simulink model "PlantModel"  (R2021b)
settings: configuration reference "MIL_Simulation_ConfigSet" (kept outside this file)
PreLoadFcn:
  | run_start;
undefined symbols (not defined in the file or in its folder): DiscIntNeverNeededParam, F, inverter_ena, J, L_d, L_q, p, Psi_p, R, U_bat
settings Model: DataDictionary=FieldOrientedControl.sldd  Creator=Markez  LastModifiedBy=Markez
settings ConfigSetRef: SourceName=MIL_Simulation_ConfigSet

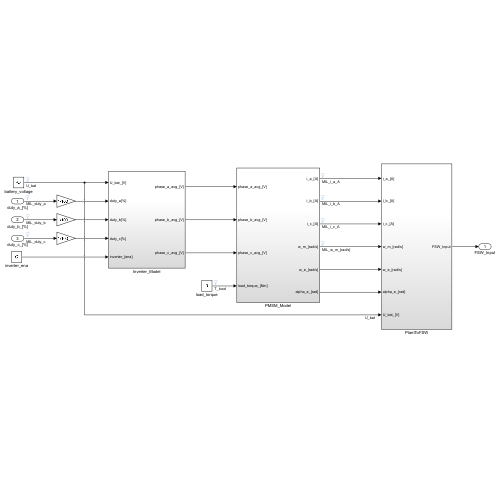
[thumbnail: Simulink's stored preview of the top-level diagram]
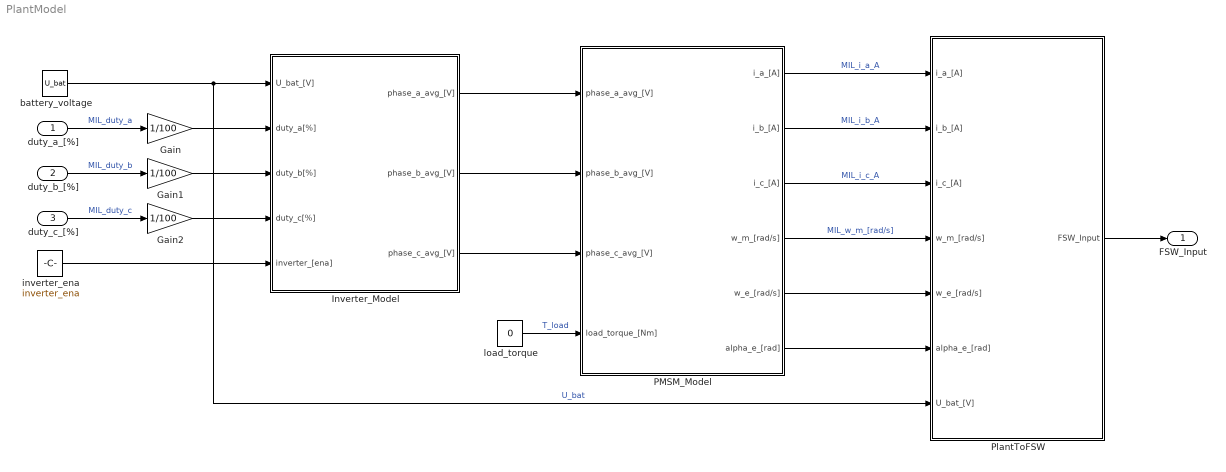
== system PlantModel ==
  duty_a_[%] : Inport
  duty_b_[%] : Inport  Port=2
  duty_c_[%] : Inport  Port=3
  Gain : Gain  Gain=1/100  RndMeth=Simplest  SaturateOnIntegerOverflow=on
  Gain1 : Gain  Gain=1/100  RndMeth=Simplest  SaturateOnIntegerOverflow=on
  Gain2 : Gain  Gain=1/100  RndMeth=Simplest  SaturateOnIntegerOverflow=on
  Inverter_Model : Subsystem
  PMSM_Model : Subsystem
  PlantToFSW : Subsystem
  battery_voltage : Constant  Value=U_bat  OutDataTypeStr=single
  inverter_ena : Constant  Value=inverter_ena  OutDataTypeStr=boolean
  load_torque : Constant  Value=0  OutDataTypeStr=single
  FSW_Input : Outport
  wires:
  PMSM_Model/3(i_c_[A]) -> PlantToFSW/3(i_c_[A])  "MIL_i_c_A"
  Gain1/1 -> Inverter_Model/3(duty_b[%])
  PlantToFSW/1(FSW_Input) -> FSW_Input/1
  PMSM_Model/6(alpha_e_[rad]) -> PlantToFSW/6(alpha_e_[rad])
  Gain2/1 -> Inverter_Model/4(duty_c[%])
  PMSM_Model/4(w_m_[rad/s]) -> PlantToFSW/4(w_m_[rad/s])  "MIL_w_m_[rad/s]"
  PMSM_Model/5(w_e_[rad/s]) -> PlantToFSW/5(w_e_[rad/s])
  inverter_ena/1 -> Inverter_Model/5(inverter_[ena])
  Gain/1 -> Inverter_Model/2(duty_a[%])
  Inverter_Model/3(phase_c_avg_[V]) -> PMSM_Model/3(phase_c_avg_[V])
  PMSM_Model/2(i_b_[A]) -> PlantToFSW/2(i_b_[A])  "MIL_i_b_A"
  duty_b_[%]/1 -> Gain1/1  "MIL_duty_b"
  load_torque/1 -> PMSM_Model/4(load_torque_[Nm])  "T_load"
  PMSM_Model/1(i_a_[A]) -> PlantToFSW/1(i_a_[A])  "MIL_i_a_A"
  Inverter_Model/2(phase_b_avg_[V]) -> PMSM_Model/2(phase_b_avg_[V])
  Inverter_Model/1(phase_a_avg_[V]) -> PMSM_Model/1(phase_a_avg_[V])
  duty_c_[%]/1 -> Gain2/1  "MIL_duty_c"
  battery_voltage/1 -> PlantToFSW/7(U_bat_[V]), Inverter_Model/1(U_bat_[V])  "U_bat"
  duty_a_[%]/1 -> Gain/1  "MIL_duty_a"

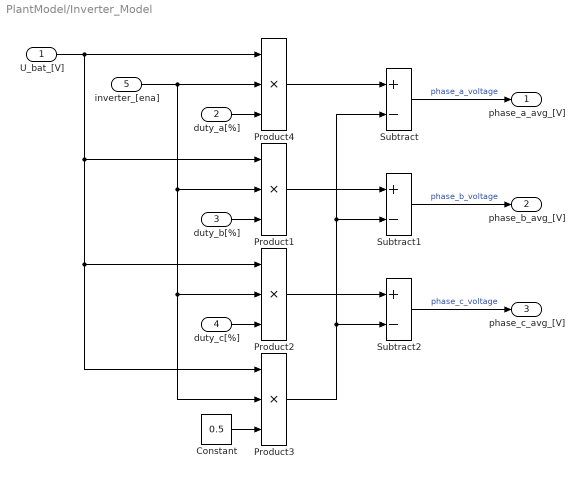
== system PlantModel/Inverter_Model ==
  U_bat_[V] : Inport
  duty_a[%] : Inport  Port=2
  duty_b[%] : Inport  Port=3
  duty_c[%] : Inport  Port=4
  inverter_[ena] : Inport  Port=5
  Constant : Constant  Value=0.5  OutDataTypeStr=single
  Product{1..4} (4 alike) : Product  Inputs=3  RndMeth=Simplest  SaturateOnIntegerOverflow=on
  Subtract : Sum  Inputs=+-  RndMeth=Simplest  SaturateOnIntegerOverflow=on
  Subtract1 : Sum  Inputs=+-  RndMeth=Simplest  SaturateOnIntegerOverflow=on
  Subtract2 : Sum  Inputs=+-  RndMeth=Simplest  SaturateOnIntegerOverflow=on
  phase_a_avg_[V] : Outport
  phase_b_avg_[V] : Outport  Port=2
  phase_c_avg_[V] : Outport  Port=3
  wires:
  U_bat_[V]/1 -> Product4/1, Product1/1, Product3/1, Product2/1
  inverter_[ena]/1 -> Product4/2, Product3/2, Product2/2, Product1/2
  duty_a[%]/1 -> Product4/3
  duty_b[%]/1 -> Product1/3
  duty_c[%]/1 -> Product2/3
  Constant/1 -> Product3/3
  Product4/1 -> Subtract/1
  Product1/1 -> Subtract1/1
  Product2/1 -> Subtract2/1
  Product3/1 -> Subtract2/2, Subtract1/2, Subtract/2
  Subtract/1 -> phase_a_avg_[V]/1  "phase_a_voltage"
  Subtract1/1 -> phase_b_avg_[V]/1  "phase_b_voltage"
  Subtract2/1 -> phase_c_avg_[V]/1  "phase_c_voltage"

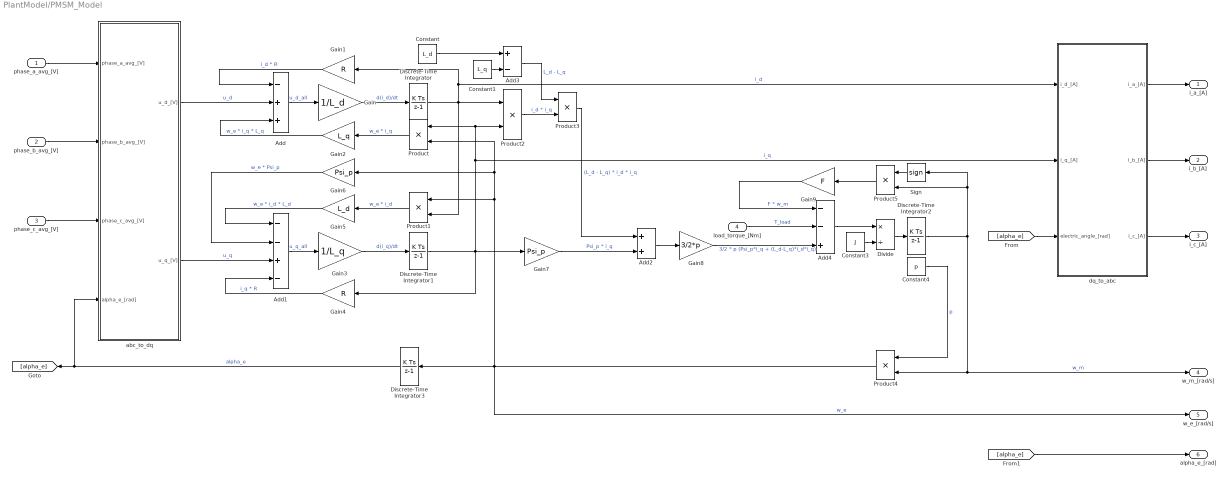
== system PlantModel/PMSM_Model ==
  phase_a_avg_[V] : Inport
  phase_b_avg_[V] : Inport  Port=2
  phase_c_avg_[V] : Inport  Port=3
  load_torque_[Nm] : Inport  Port=4
  Add : Sum  Inputs=-++  RndMeth=Simplest  SaturateOnIntegerOverflow=on
  Add1 : Sum  Inputs=--+-  RndMeth=Simplest  SaturateOnIntegerOverflow=on
  Add2 : Sum  RndMeth=Simplest  SaturateOnIntegerOverflow=on
  Add3 : Sum  Inputs=+-  RndMeth=Simplest  SaturateOnIntegerOverflow=on
  Add4 : Sum  Inputs=--+  RndMeth=Simplest  SaturateOnIntegerOverflow=on
  Constant : Constant  Value=L_d  OutDataTypeStr=single
  Constant1 : Constant  Value=L_q  OutDataTypeStr=single
  Constant3 : Constant  Value=J  OutDataTypeStr=single
  Constant4 : Constant  Value=p  OutDataTypeStr=single
  Discrete-Time Integrator : DiscreteIntegrator  gainval=L_d/R  SampleTime=-1  RndMeth=Simplest  SaturateOnIntegerOverflow=on  ICPrevOutput=DiscIntNeverNeededParam  ICPrevScaledInput=DiscIntNeverNeededParam
  Discrete-Time Integrator1 : DiscreteIntegrator  gainval=L_q/R  SampleTime=-1  RndMeth=Simplest  SaturateOnIntegerOverflow=on  ICPrevOutput=DiscIntNeverNeededParam  ICPrevScaledInput=DiscIntNeverNeededParam
  Discrete-Time Integrator2 : DiscreteIntegrator  SampleTime=-1  RndMeth=Simplest  SaturateOnIntegerOverflow=on  ICPrevOutput=DiscIntNeverNeededParam  ICPrevScaledInput=DiscIntNeverNeededParam
  Discrete-Time Integrator3 : DiscreteIntegrator  SampleTime=-1  RndMeth=Simplest  SaturateOnIntegerOverflow=on  ICPrevOutput=DiscIntNeverNeededParam  ICPrevScaledInput=DiscIntNeverNeededParam
  Divide : Product  Inputs=*/  RndMeth=Simplest  SaturateOnIntegerOverflow=on
  Gain : Gain  Gain=1/L_d  RndMeth=Simplest  SaturateOnIntegerOverflow=on
  Gain1 : Gain  Gain=R  RndMeth=Simplest  SaturateOnIntegerOverflow=on
  Gain2 : Gain  Gain=L_q  RndMeth=Simplest  SaturateOnIntegerOverflow=on
  Gain3 : Gain  Gain=1/L_q  RndMeth=Simplest  SaturateOnIntegerOverflow=on
  Gain4 : Gain  Gain=R  RndMeth=Simplest  SaturateOnIntegerOverflow=on
  Gain5 : Gain  Gain=L_d  RndMeth=Simplest  SaturateOnIntegerOverflow=on
  Gain6 : Gain  Gain=Psi_p  RndMeth=Simplest  SaturateOnIntegerOverflow=on
  Gain7 : Gain  Gain=Psi_p  RndMeth=Simplest  SaturateOnIntegerOverflow=on
  Gain8 : Gain  Gain=3/2*p  RndMeth=Simplest  SaturateOnIntegerOverflow=on
  Gain9 : Gain  Gain=F  RndMeth=Simplest  SaturateOnIntegerOverflow=on
  Product{,1..5} (6 alike) : Product  RndMeth=Simplest  SaturateOnIntegerOverflow=on
  Sign : Signum
  abc_to_dq : Subsystem
  dq_to_abc : Subsystem
  i_a_[A] : Outport
  i_b_[A] : Outport  Port=2
  i_c_[A] : Outport  Port=3
  w_m_[rad/s] : Outport  Port=4
  w_e_[rad/s] : Outport  Port=5
  alpha_e_[rad] : Outport  Port=6
  wires:
  phase_a_avg_[V]/1 -> abc_to_dq/1(phase_a_avg_[V])
  phase_b_avg_[V]/1 -> abc_to_dq/2(phase_b_avg_[V])
  phase_c_avg_[V]/1 -> abc_to_dq/3(phase_c_avg_[V])
  abc_to_dq/1(u_d_[V]) -> Add/2  "u_d"
  Add/1 -> Gain/1  "u_d_all"
  Gain/1 -> Discrete-Time Integrator/1  "d(i_d)/dt"
  Discrete-Time Integrator/1 -> Product2/1, Product1/2, Gain1/1, dq_to_abc/1(i_d_[A])  "i_d"
  Gain1/1 -> Add/1  "i_d * R"
  Gain2/1 -> Add/3  "w_e * i_q * L_q"
  Product/1 -> Gain2/1  "w_e * i_q"
  Gain3/1 -> Discrete-Time Integrator1/1  "d(i_q)/dt"
  Add1/1 -> Gain3/1  "u_q_all"
  Product1/1 -> Gain5/1  "w_e * i_d"
  Discrete-Time Integrator1/1 -> Gain7/1, Product2/2, Product/1, dq_to_abc/2(i_q_[A]), Gain4/1  "i_q"
  Gain4/1 -> Add1/4  "i_q * R"
  abc_to_dq/2(u_q_[V]) -> Add1/3  "u_q"
  Gain5/1 -> Add1/1  "w_e * i_d * L_d"
  Gain6/1 -> Add1/2  "w_e * Psi_p"
  Gain7/1 -> Add2/2  "Psi_p * i_q"
  Constant/1 -> Add3/1
  Constant1/1 -> Add3/2
  Add3/1 -> Product3/1  "L_d - L_q"
  Product2/1 -> Product3/2  "i_d * i_q"
  Product3/1 -> Add2/1  "(L_d - L_q) * i_d * i_q"
  Add2/1 -> Gain8/1
  Gain8/1 -> Add4/3  "3/2 * p (Psi_p*i_q + (L_d-L_q)*i_d*i_q)"
  load_torque_[Nm]/1 -> Add4/2  "T_load"
  Gain9/1 -> Add4/1  "F * w_m"
  Add4/1 -> Divide/1
  Constant3/1 -> Divide/2
  Divide/1 -> Discrete-Time Integrator2/1
  Discrete-Time Integrator2/1 -> Product5/2, Sign/1, w_m_[rad/s]/1, Product4/2  "w_m"
  Product4/1 -> w_e_[rad/s]/1, Product/2, Gain6/1, Product1/1, Discrete-Time Integrator3/1  "w_e"
  Discrete-Time Integrator3/1 -> [alpha_e], abc_to_dq/4(alpha_e_[rad])  "alpha_e"
  Constant4/1 -> Product4/1  "p"
  [alpha_e] -> dq_to_abc/3(electric_angle_[rad])
  dq_to_abc/1(i_a_[A]) -> i_a_[A]/1
  dq_to_abc/3(i_c_[A]) -> i_c_[A]/1
  dq_to_abc/2(i_b_[A]) -> i_b_[A]/1
  [alpha_e] -> alpha_e_[rad]/1
  Sign/1 -> Product5/1
  Product5/1 -> Gain9/1

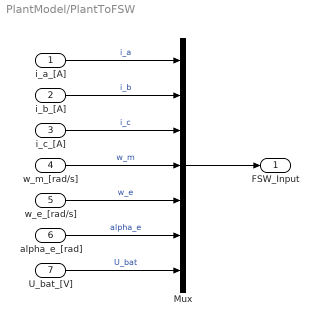
== system PlantModel/PlantToFSW ==
  i_a_[A] : Inport
  i_b_[A] : Inport  Port=2
  i_c_[A] : Inport  Port=3
  w_m_[rad/s] : Inport  Port=4
  w_e_[rad/s] : Inport  Port=5
  alpha_e_[rad] : Inport  Port=6
  U_bat_[V] : Inport  Port=7
  Mux : Mux  Inputs=7
  FSW_Input : Outport
  wires:
  Mux/1 -> FSW_Input/1
  i_a_[A]/1 -> Mux/1  "i_a"
  i_b_[A]/1 -> Mux/2  "i_b"
  U_bat_[V]/1 -> Mux/7  "U_bat"
  w_m_[rad/s]/1 -> Mux/4  "w_m"
  i_c_[A]/1 -> Mux/3  "i_c"
  alpha_e_[rad]/1 -> Mux/6  "alpha_e"
  w_e_[rad/s]/1 -> Mux/5  "w_e"

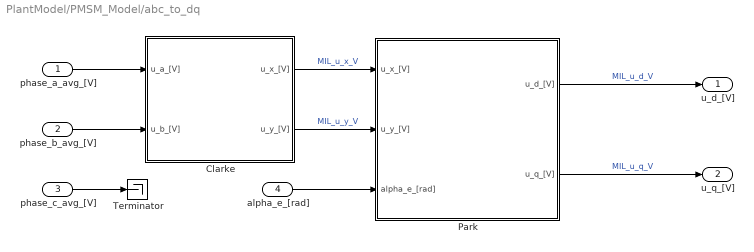
== system PlantModel/PMSM_Model/abc_to_dq ==
  phase_a_avg_[V] : Inport
  phase_b_avg_[V] : Inport  Port=2
  phase_c_avg_[V] : Inport  Port=3
  alpha_e_[rad] : Inport  Port=4
  Clarke : Subsystem
  Park : Subsystem
  Terminator : Terminator
  u_d_[V] : Outport
  u_q_[V] : Outport  Port=2
  wires:
  phase_a_avg_[V]/1 -> Clarke/1(u_a_[V])
  phase_b_avg_[V]/1 -> Clarke/2(u_b_[V])
  Clarke/1(u_x_[V]) -> Park/1(u_x_[V])  "MIL_u_x_V"
  Clarke/2(u_y_[V]) -> Park/2(u_y_[V])  "MIL_u_y_V"
  alpha_e_[rad]/1 -> Park/3(alpha_e_[rad])
  Park/1(u_d_[V]) -> u_d_[V]/1  "MIL_u_d_V"
  Park/2(u_q_[V]) -> u_q_[V]/1  "MIL_u_q_V"
  phase_c_avg_[V]/1 -> Terminator/1

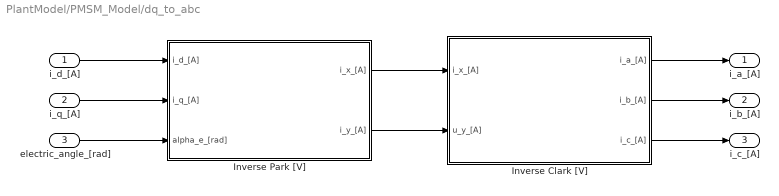
== system PlantModel/PMSM_Model/dq_to_abc ==
  i_d_[A] : Inport
  i_q_[A] : Inport  Port=2
  electric_angle_[rad] : Inport  Port=3
  Inverse Clark [V] : Subsystem
  Inverse Park [V] : Subsystem
  i_a_[A] : Outport
  i_b_[A] : Outport  Port=2
  i_c_[A] : Outport  Port=3
  wires:
  i_d_[A]/1 -> Inverse Park [V]/1(i_d_[A])
  i_q_[A]/1 -> Inverse Park [V]/2(i_q_[A])
  electric_angle_[rad]/1 -> Inverse Park [V]/3(alpha_e_[rad])
  Inverse Park [V]/1(i_x_[A]) -> Inverse Clark [V]/1(i_x_[A])
  Inverse Park [V]/2(i_y_[A]) -> Inverse Clark [V]/2(u_y_[A])
  Inverse Clark [V]/1(i_a_[A]) -> i_a_[A]/1
  Inverse Clark [V]/3(i_c_[A]) -> i_c_[A]/1
  Inverse Clark [V]/2(i_b_[A]) -> i_b_[A]/1

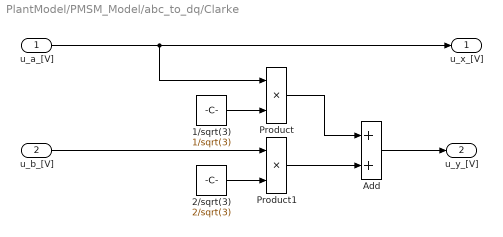
== system PlantModel/PMSM_Model/abc_to_dq/Clarke ==
  u_a_[V] : Inport
  u_b_[V] : Inport  Port=2
  1/sqrt(3) : Constant  Value=1/sqrt(3)  OutDataTypeStr=single
  2/sqrt(3) : Constant  Value=2/sqrt(3)  OutDataTypeStr=single
  Add : Sum  RndMeth=Simplest  SaturateOnIntegerOverflow=on
  Product : Product  RndMeth=Simplest  SaturateOnIntegerOverflow=on
  Product1 : Product  RndMeth=Simplest  SaturateOnIntegerOverflow=on
  u_x_[V] : Outport
  u_y_[V] : Outport  Port=2
  wires:
  u_a_[V]/1 -> u_x_[V]/1, Product/1
  1/sqrt(3)/1 -> Product/2
  2/sqrt(3)/1 -> Product1/2
  u_b_[V]/1 -> Product1/1
  Product1/1 -> Add/2
  Product/1 -> Add/1
  Add/1 -> u_y_[V]/1

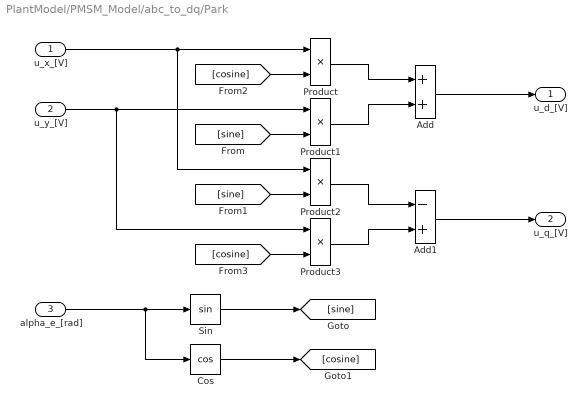
== system PlantModel/PMSM_Model/abc_to_dq/Park ==
  u_x_[V] : Inport
  u_y_[V] : Inport  Port=2
  alpha_e_[rad] : Inport  Port=3
  Add : Sum  RndMeth=Simplest  SaturateOnIntegerOverflow=on
  Add1 : Sum  Inputs=-+  RndMeth=Simplest  SaturateOnIntegerOverflow=on
  Cos : Trigonometry  Operator=cos
  Product{,1..3} (4 alike) : Product  RndMeth=Simplest  SaturateOnIntegerOverflow=on
  Sin : Trigonometry
  u_d_[V] : Outport
  u_q_[V] : Outport  Port=2
  wires:
  alpha_e_[rad]/1 -> Cos/1, Sin/1
  Sin/1 -> [sine]
  Cos/1 -> [cosine]
  u_x_[V]/1 -> Product2/1, Product/1
  u_y_[V]/1 -> Product3/1, Product1/1
  [sine] -> Product1/2
  [sine] -> Product2/2
  [cosine] -> Product/2
  [cosine] -> Product3/2
  Product/1 -> Add/1
  Product1/1 -> Add/2
  Add/1 -> u_d_[V]/1
  Product2/1 -> Add1/1
  Product3/1 -> Add1/2
  Add1/1 -> u_q_[V]/1

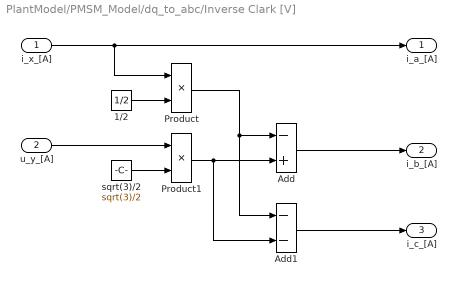
== system PlantModel/PMSM_Model/dq_to_abc/Inverse Clark [V] ==
  i_x_[A] : Inport
  u_y_[A] : Inport  Port=2
  1/2 : Constant  Value=1/2  OutDataTypeStr=single
  Add : Sum  Inputs=-+  RndMeth=Simplest  SaturateOnIntegerOverflow=on
  Add1 : Sum  Inputs=--  RndMeth=Simplest  SaturateOnIntegerOverflow=on
  Product : Product  RndMeth=Simplest  SaturateOnIntegerOverflow=on
  Product1 : Product  RndMeth=Simplest  SaturateOnIntegerOverflow=on
  sqrt(3)/2 : Constant  Value=sqrt(3)/2  OutDataTypeStr=single
  i_a_[A] : Outport
  i_b_[A] : Outport  Port=2
  i_c_[A] : Outport  Port=3
  wires:
  i_x_[A]/1 -> i_a_[A]/1, Product/1
  1/2/1 -> Product/2
  sqrt(3)/2/1 -> Product1/2
  u_y_[A]/1 -> Product1/1
  Product/1 -> Add1/1, Add/1
  Product1/1 -> Add1/2, Add/2
  Add/1 -> i_b_[A]/1
  Add1/1 -> i_c_[A]/1

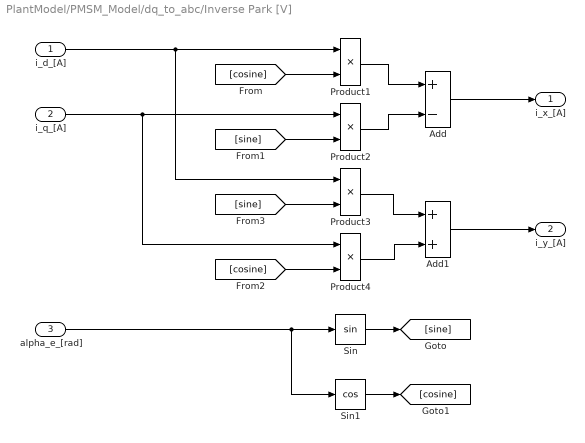
== system PlantModel/PMSM_Model/dq_to_abc/Inverse Park [V] ==
  i_d_[A] : Inport
  i_q_[A] : Inport  Port=2
  alpha_e_[rad] : Inport  Port=3
  Add : Sum  Inputs=+-  RndMeth=Simplest  SaturateOnIntegerOverflow=on
  Add1 : Sum  RndMeth=Simplest  SaturateOnIntegerOverflow=on
  Product{1..4} (4 alike) : Product  RndMeth=Simplest  SaturateOnIntegerOverflow=on
  Sin : Trigonometry  NumberOfDataPoints=256
  Sin1 : Trigonometry  Operator=cos  NumberOfDataPoints=256
  i_x_[A] : Outport
  i_y_[A] : Outport  Port=2
  wires:
  Sin/1 -> [sine]
  [cosine] -> Product1/2
  i_d_[A]/1 -> Product3/1, Product1/1
  [sine] -> Product2/2
  i_q_[A]/1 -> Product4/1, Product2/1
  Product1/1 -> Add/1
  Product2/1 -> Add/2
  Add/1 -> i_x_[A]/1
  Product3/1 -> Add1/1
  Product4/1 -> Add1/2
  Add1/1 -> i_y_[A]/1
  alpha_e_[rad]/1 -> Sin1/1, Sin/1
  Sin1/1 -> [cosine]
  [sine] -> Product3/2
  [cosine] -> Product4/2
